simulink model "aimant_permanent_tf"  (R2019a)
settings: Solver=VariableStepAuto  StartTime=0.0  StopTime=10.0  RelTol=1e-3
undefined symbols (not defined in the file): Bm, J, Kv, LAA, ra, Tl, Va
settings Model: Creator=azizi  LastModifiedBy=azizi

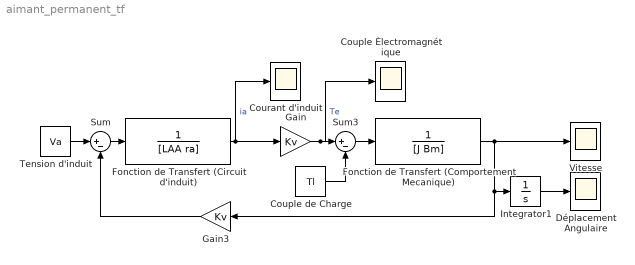
== system aimant_permanent_tf ==
  Couple de Charge : Constant  Value=Tl
  Couple Èlectromagnétique : Scope
  Courant d'induit : Scope
  Déplacement Angulaire : Scope
  Fonction de Transfert (Circuit d'induit) : TransferFcn  Denominator=[LAA ra]
  Fonction de Transfert (Comportement Mecanique) : TransferFcn  Denominator=[J Bm]
  Gain : Gain  Gain=Kv
  Gain3 : Gain  Gain=Kv
  Integrator1 : Integrator
  Sum : Sum  Inputs=|+-
  Sum3 : Sum  Inputs=|+-
  Tension d'induit : Constant  Value=Va
  Vitesse : Scope
  wires:
  Sum/1 -> Fonction de Transfert (Circuit d'induit)/1
  Tension d'induit/1 -> Sum/1
  Fonction de Transfert (Comportement Mecanique)/1 -> Vitesse/1, Integrator1/1, Gain3/1
  Gain/1 -> Couple Èlectromagnétique/1, Sum3/1  "Te"
  Integrator1/1 -> Déplacement Angulaire/1
  Sum3/1 -> Fonction de Transfert (Comportement Mecanique)/1
  Fonction de Transfert (Circuit d'induit)/1 -> Courant d'induit/1, Gain/1  "ia"
  Couple de Charge/1 -> Sum3/2
  Gain3/1 -> Sum/2
